simulink model "experiment_toplevel"  (R2016a)
settings: Solver=ode15s  StartTime=0.0  StopTime=20  MaxStep=1e-2  RelTol=1e-4
PreLoadFcn:
  | minitaurParameters
values from neighbouring files (symbols this model uses):
  angular_ctrl_d = 1    [minitaurParameters.m]
  angular_ctrl_i = 1    [minitaurParameters.m]
  angular_ctrl_p = 100    [minitaurParameters.m]
  enc_zero_IA = -1.25*pi    (= -3.92699081699)    [minitaurParameters.m]
  enc_zero_IB = -0.25*pi    (= -0.785398163397)    [minitaurParameters.m]
  enc_zero_IIA = 1.25*pi    (= 3.92699081699)    [minitaurParameters.m]
  enc_zero_IIB = 1.25*pi    (= 3.92699081699)    [minitaurParameters.m]
  enc_zero_IIIA = 0.5*pi    (= 1.57079632679)    [minitaurParameters.m]
  enc_zero_IIIB = 1.5*pi    (= 4.71238898038)    [minitaurParameters.m]
  enc_zero_IVA = -0.25*pi    (= -0.785398163397)    [minitaurParameters.m]
  enc_zero_IVB = 0.5*pi    (= 1.57079632679)    [minitaurParameters.m]
  fore_lag = fore_lag_vals(j)    [experiment1.m]    (also in experiment1_parfor_accelerator.m = 0; minitaurParameters.m = 0.45)
  ground_frame_depth = 0.5    [minitaurParameters.m]
  ground_length = 100    [minitaurParameters.m]
  ground_width = 10    [minitaurParameters.m]
  init_theta_IA = -pi/4    (= -0.785398163397)    [minitaurParameters.m]
  init_theta_IB = pi/4    (= 0.785398163397)    [minitaurParameters.m]
  init_theta_IIA = -pi/4    (= -0.785398163397)    [minitaurParameters.m]
  init_theta_IIB = pi/4    (= 0.785398163397)    [minitaurParameters.m]
  init_theta_IIIA = -pi/4    (= -0.785398163397)    [minitaurParameters.m]
  init_theta_IIIB = pi/4    (= 0.785398163397)    [minitaurParameters.m]
  init_theta_IVA = -pi/4    (= -0.785398163397)    [minitaurParameters.m]
  init_theta_IVB = pi/4    (= 0.785398163397)    [minitaurParameters.m]
  l1 = 100e-3    (= 0.1)    [minitaurParameters.m]
  l2 = 200e-3    (= 0.2)    [minitaurParameters.m]
  leg_joint_radius = 3e-3    (= 0.003)    [minitaurParameters.m]
  lr_sync = 1    [experiment1.m]    (also in experiment1_parfor_accelerator.m; minitaurParameters.m = 0)
  model = 'experiment_toplevel'    [experiment1_parfor_accelerator.m]
  period = period_vals(i)    [experiment1.m]    (also in experiment1_parfor_accelerator.m = 1.5; minitaurParameters.m = 0.33)
  phi_0 = 0.5*asin(l1/l2)    [experiment1.m]    (also in experiment1_parfor_accelerator.m; minitaurParameters.m)
  r_0 = l2    [experiment1.m]    (also in experiment1_parfor_accelerator.m; minitaurParameters.m = 0.2)
  r_x = 0.3*l1    [experiment1.m]    (also in experiment1_parfor_accelerator.m = 0.5*l1; minitaurParameters.m = 0.05)
  r_y = 0.2*l1    [experiment1.m]    (also in experiment1_parfor_accelerator.m = 0.3*l1; minitaurParameters.m = 0.03)
  radial_ctrl_d = 1    [minitaurParameters.m]
  radial_ctrl_i = 1    [minitaurParameters.m]
  radial_ctrl_p = 80    [minitaurParameters.m]
  safety_limit = 10e-3    (= 0.01)    [minitaurParameters.m]
undefined symbols (not defined in the file or in its folder): Axis, Fn, minitaurParams, r_stance, r_swing, stance_frac, X, Y, Z
undefined symbols (not defined in the file): leg_joint_fric_bw, leg_joint_mu_k, leg_joint_mu_s, leg_joint_vel_thresh, motor_kt, motor_kv, motor_r, motor_torque_sat
libraries: sm_lib x453, fl_lib x132, nesl_utility x31, Contact_Forces_Lib x28, simulink x19
(part 1 of 13)
settings Model: TunableVars=fore_lag,lr_sync,period  TunableVarsStorageClass=Auto,Auto,Auto  TunableVarsTypeQualifier=,,  Creator=Alexander  LastModifiedBy=Joe
settings SolverCC: MaxOrder=3  AlgebraicLoopSolver=LineSearch
settings DataIOCC: SaveFormat=StructureWithTime  SaveOutput=off  DSMLogging=off  SaveTime=off  SignalLoggingName=output
settings OptimizationCC: DefaultParameterBehavior=Inlined  InlineInvariantSignals=on  EfficientFloat2IntCast=on  EfficientMapNaN2IntZero=off  AccelVerboseBuild=on
settings DebuggingCC: ReadBeforeWriteMsg=DisableAll  WriteAfterWriteMsg=DisableAll  WriteAfterReadMsg=DisableAll  MultiTaskDSMMsg=none  StrictBusMsg=ErrorOnBusTreatedAsVector
settings HardwareCC: TargetBitPerPointer=64  TargetLongLongMode=on  TargetIntDivRoundTo=Zero  TargetEndianess=LittleEndian  TargetWordSize=64  TargetHWDeviceType=MATLAB Host  ProdEqTarget=off
settings ModelReferenceCC: UpdateModelReferenceTargets=IfOutOfDate  ModelReferenceMinAlgLoopOccurrences=on
settings SFSimCC: SFSimEcho=off  SimBuildMode=sf_nonincremental_build
settings RTWCC: SystemTargetFile=rsim.tlc  TemplateMakefile=rsim_default_tmf  Description=Rapid Simulation Target  Toolchain=MinGW64 v4.x | gmake (64-bit Windows)
settings CodeAppCC: GenerateComments=off  SimulinkBlockComments=off
settings RSimTargetCC: ERTMultiwordTypeDef=System defined  ERTMultiwordLength=256  ConcurrentExecutionCompliant=off  GeneratePreprocessorConditionals=Use local settings  SupportNonFinite=off
settings DiagnosticsConfigSet: SimMechanicsRigidlyBoundBlock=none
settings ExplorerConfigSet: InternalSimMechanicsExplorerSettings="<ExplorerConfiguration><canonicalview>default</canonicalview><AnimationSetting><BasePlaybackSpeed>1.0</BasePlaybackSpeed><PlaybackSpeedFactor>0.015625</PlaybackSpeedFactor></AnimationSetting><TilePanel><TileInfo><Tiles Columns=\"1\" Count=\"1\" Rows=\"1\"><Column Left=\"2\" Weight=\"1\"/><Column Left=\"1404\"/><Row Top=\"2\" Weight=\"1\"/><Row Top=\"894\"/><Tile Height=\"1\" Width=\"1\" X=\"0\" Y=\"0\"/></Tiles></TileInfo><SceneInfo><SceneViewer><BGColor><R>1</R><G>1</G><B>1</B></BGColor><Camera><DoPerspective>off</DoPerspective><Position><X>51.2033483715938971</X><Y>-47.1572080477410083</Y><Z>0.726349227559124011</Z></Position><Center><X>-1.27720243625617513e-06</X><Y>-47.1572080477410083</Y><Z>0.726349227559124011</Z></Center><Up><X>-0</X><Y>0</Y><Z>1</Z></Up><ViewLimDist>1</ViewLimDist><YLim>0.527619672638390491</YLim><XLim>0.832360366914244643</XLim></Camera></SceneViewer></SceneInfo></TilePanel><MechEditorPanel><Cameras><Camera><Id>Camera1</Id><Value><Name>Camera1</Name><NativeCamera><PositionKeyframeSet><Keyframe><Time>+0.0000000000000000e+00</Time><Value><X>+1.6016183665152193e+00</X><Y>-4.6009050514178448e+01</Y><Z>+8.6329844289606328e-01</Z></Value></Keyframe></PositionKeyframeSet><CenterKeyframeSet><Keyframe><Time>+0.0000000000000000e+00</Time><Value><X>+4.1998902890613099e-01</X><Y>-4.6399928223387391e+01</Y><Z>+4.9999520687549426e-01</Z></Value></Keyframe></CenterKeyframeSet><UpVectorKeyframeSet><Keyframe><Time>+0.0000000000000000e+00</Time><Value><X>-2.4497970609361264e-01</X><Y>-1.4974251475434000e-01</Y><Z>+9.5789463036251210e-01</Z></Value></Keyframe></UpVectorKeyframeSet></NativeCamera></Value></Camera></Cameras><GfxPanelCameraMap/></MechEditorPanel></ExplorerConfiguration>"

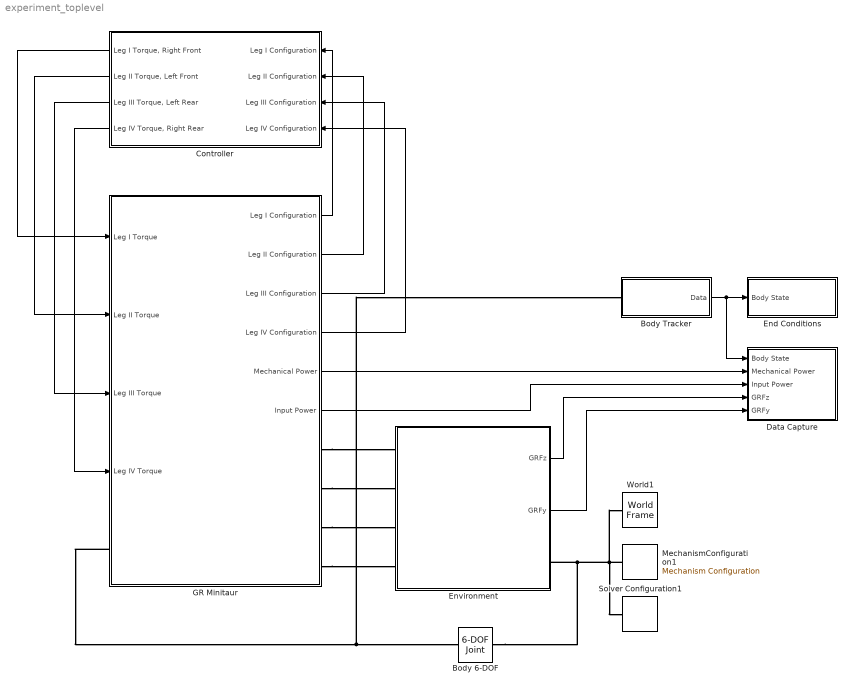
== system experiment_toplevel ==
  Body 6-DOF : sm_lib/Joints/6-DOF Joint  SenseConstraintForce=off  SenseConstraintForceX=off  SenseConstraintForceY=off  SenseConstraintForceZ=off  SenseConstraintTorque=off  SenseConstraintTorqueX=off  SenseConstraintTorqueY=off  SenseConstraintTorqueZ=off  SenseTotalForce=off  SenseTotalForceX=off  SenseTotalForceY=off  SenseTotalForceZ=off  SenseTotalTorque=off  SenseTotalTorqueX=off  SenseTotalTorqueY=off  SenseTotalTorqueZ=off  CompositeWrenchDir=FollowerOnBase  CompositeWrenchFrame=BaseFrame  PxEquilibriumPosition=0  PxEquilibriumPositionUnits=m  PxSpringStiffness=0  PxSpringStiffnessUnits=N/m  PxDampingCoefficient=0  PxDampingCoefficientUnits=N/(m/s)  PxTorqueActuationMode=NoTorque  PxMotionActuationMode=ComputedMotion  PxSensePosition=off  PxSenseVelocity=off  PxSenseAcceleration=off  PxSenseTorqueForce=off  PxPositionTargetSpecify=on  PxPositionTargetPriority=High  PxPositionTargetValue=init_x  PxPositionTargetValueUnits=m  PxVelocityTargetSpecify=off  PxVelocityTargetPriority=High  PxVelocityTargetValue=0  PxVelocityTargetValueUnits=m/s  PyEquilibriumPosition=0  PyEquilibriumPositionUnits=m  PySpringStiffness=0  PySpringStiffnessUnits=N/m  PyDampingCoefficient=0  PyDampingCoefficientUnits=N/(m/s)  PyTorqueActuationMode=NoTorque  PyMotionActuationMode=ComputedMotion  PySensePosition=off  PySenseVelocity=off  PySenseAcceleration=off  PySenseTorqueForce=off  PyPositionTargetSpecify=on  PyPositionTargetPriority=High  PyPositionTargetValue=init_y  PyPositionTargetValueUnits=m  PyVelocityTargetSpecify=off  PyVelocityTargetPriority=High  PyVelocityTargetValue=0  PyVelocityTargetValueUnits=m/s  PzEquilibriumPosition=1  PzEquilibriumPositionUnits=m  PzSpringStiffness=0  PzSpringStiffnessUnits=N/m  PzDampingCoefficient=0  PzDampingCoefficientUnits=N/(m/s)  PzTorqueActuationMode=NoTorque  PzMotionActuationMode=ComputedMotion  PzSensePosition=off  PzSenseVelocity=off  PzSenseAcceleration=off  PzSenseTorqueForce=off  PzPositionTargetSpecify=on  PzPositionTargetPriority=High  PzPositionTargetValue=init_z  PzPositionTargetValueUnits=m  PzVelocityTargetSpecify=off  PzVelocityTargetPriority=High  PzVelocityTargetValue=0  PzVelocityTargetValueUnits=m/s  SphDefPosRotationMethod=None  SphDefPosRotationAngleUnits=deg  SphDefPosRotationStandardAxis=+Z  SphDefPosRotationAngle=0.0  SphDefPosRotationArbitraryAxis=[0 0 1]  SphDefPosFollAlignAxisA=+X  SphDefPosBaseAlignAxisA=+Y  SphDefPosFollAlignAxisB=+Y  SphDefPosBaseAlignAxisB=+Z  SphDefPosRotationSequenceAxes=FollowerAxes  SphDefPosRotationSequence=XYX  SphDefPosRotationSequenceAngles=[0 0 0]  SphDefPosRotationSequenceAnglesUnits=deg  SphDefPosRotationMatrix=[1 0 0; 0 1 0; 0 0 1]  SphEqPosRotationMethod=None  SphEqPosRotationAngleUnits=deg  SphEqPosRotationStandardAxis=+Z  SphEqPosRotationAngle=0.0  SphEqPosRotationArbitraryAxis=[0 0 1]  SphEqPosFollAlignAxisA=+X  SphEqPosBaseAlignAxisA=+Y  SphEqPosFollAlignAxisB=+Y  SphEqPosBaseAlignAxisB=+Z  SphEqPosRotationSequenceAxes=FollowerAxes  SphEqPosRotationSequence=XYX  SphEqPosRotationSequenceAngles=[0 0 0]  SphEqPosRotationSequenceAnglesUnits=deg  SphEqPosRotationMatrix=[1 0 0; 0 1 0; 0 0 1]  SphSpringStiffness=0  SphSpringStiffnessUnits=N*m/deg  SphDampingCoefficient=0  SphDampingCoefficientUnits=N*m/(deg/s)  SphActuateTorqueX=off  SphActuateTorqueY=off  SphActuateTorqueZ=off  SphActuateTorque=off  SphTorqueActuationMode=NoTorque  SphMotionActuationMode=ComputedMotion  SphActuationFrame=BaseFrame  SphSensePosition=off  SphSenseVelocityX=off  SphSenseVelocityY=off  SphSenseVelocityZ=off  SphSenseVelocity=off  SphSenseAccelerationX=off  SphSenseAccelerationY=off  SphSenseAccelerationZ=off  SphSenseAcceleration=off  SphSenseTorqueX=off  SphSenseTorqueY=off  SphSenseTorqueZ=off  SphSenseTorqueForce=off  SphSensingFrame=BaseFrame  SphPositionTargetRotationMethod=RotationSequence  SphPositionTargetRotationAngleUnits=deg  SphPositionTargetRotationStandardAxis=+Z  SphPositionTargetRotationAngle=0.0  SphPositionTargetRotationArbitraryAxis=[0 0 1]  SphPositionTargetFollAlignAxisA=+X  SphPositionTargetBaseAlignAxisA=+Y  SphPositionTargetFollAlignAxisB=+Y  SphPositionTargetBaseAlignAxisB=+Z  SphPositionTargetRotationSequenceAxes=BaseAxes  SphPositionTargetRotationSequence=XZX  SphPositionTargetRotationSequenceAngles=init_rot_xzx  SphPositionTargetRotationSequenceAnglesUnits=deg  SphPositionTargetRotationMatrix=[1 0 0; 0 1 0; 0 0 1]  SphPositionTargetSpecify=on  SphPositionTargetPriority=High  SphVelocityTargetValue=[0 0 0]  SphVelocityTargetValueUnits=deg/s  SphVelocityTargetSpecify=off  SphVelocityTargetPriority=High  SphVelocityTargetInFollowerFrame=on
  Body Tracker : Subsystem
  Controller : Subsystem
  Data Capture : Subsystem
  End Conditions : Subsystem
  Environment : Subsystem
  GR Minitaur : Subsystem
  MechanismConfiguration1 : sm_lib/Utilities/Mechanism Configuration  UniformGravity=Constant  GravityVector="[0  0 -9.81]"  GravityUnits=m/s^2  LinearizationDelta=0.001
  Solver Configuration1 : nesl_utility/Solver Configuration  PhysicalDomain=network_engine_domain  SubClassName=solver  LeftPortType=input  RightPortType=generic  Accelerate=off  Tones=[]  Harmonics=[]  SimulateNoise=off  Profile=off  UseLocalSampling=off  EnableSwitchedLinearOptims=on  FrequencyDomain=off  UseCCode=off  RelTol=0.001  AbsTol=1e-06  MinStep=1e-09  ToWorkspace=off  RevertToSquareIcSolve=off  NumHomotopyIterations=100  PhasorMode=off  PhasorModeNumHarmonics=1  OverrideAbsTol=off  DoDC=off  ResidualTolerance=1e-09  UseLocalSolver=off  LocalSolverChoice=NE_BACKWARD_EULER_ADVANCER  LocalSolverSampleTime=0.001  DoFixedCost=off  MaxNonlinIter=3  MaxModeIter=2  LinearAlgebra=Sparse  DelaysMemoryBudget=1024  AutomaticFiltering=on  FilteringTimeConstant=0.001
  World1 : sm_lib/Frames and Transforms/World Frame
  wires:
  GR Minitaur/1(Leg I Configuration) -> Controller/1(Leg I Configuration)
  GR Minitaur/2(Leg II Configuration) -> Controller/2(Leg II Configuration)
  GR Minitaur/4(Leg IV Configuration) -> Controller/4(Leg IV Configuration)
  Controller/4("Leg IV Torque, Right Rear") -> GR Minitaur/4(Leg IV Torque)
  Controller/3("Leg III Torque, Left Rear") -> GR Minitaur/3(Leg III Torque)
  Controller/2("Leg II Torque, Left Front") -> GR Minitaur/2(Leg II Torque)
  Controller/1("Leg I Torque, Right Front") -> GR Minitaur/1(Leg I Torque)
  Body Tracker/1(Data) -> Data Capture/1(Body State), End Conditions/1(Body State)
  GR Minitaur/5(Mechanical Power) -> Data Capture/2(Mechanical Power)
  GR Minitaur/6(Input Power) -> Data Capture/3(Input Power)
  Environment/1(GRFz) -> Data Capture/4(GRFz)
  Environment/2(GRFy) -> Data Capture/5(GRFy)
  GR Minitaur/3(Leg III Configuration) -> Controller/3(Leg III Configuration)
  connections:
  MechanismConfiguration1/RConn1 -- Solver Configuration1/RConn1 -- Environment/RConn1 -- Body 6-DOF/LConn1 -- World1/RConn1
  GR Minitaur/RConn4 -- Environment/LConn4
  GR Minitaur/RConn3 -- Environment/LConn3
  GR Minitaur/RConn2 -- Environment/LConn2
  GR Minitaur/RConn1 -- Environment/LConn1
  GR Minitaur/LConn1 -- Body Tracker/LConn1 -- Body 6-DOF/RConn1

== system experiment_toplevel/Body Tracker ==
  Mux : Mux  Inputs=6
  PS-Simulink Converter : nesl_utility/PS-Simulink Converter  PhysicalDomain=network_engine_domain  SubClassName=ps_output  LeftPortType=input  RightPortType=output  PseudoPeriodic=off  Frequencies=[]  Unit=m  AffineConversion=off
  PS-Simulink Converter1 : nesl_utility/PS-Simulink Converter  PhysicalDomain=network_engine_domain  SubClassName=ps_output  LeftPortType=input  RightPortType=output  PseudoPeriodic=off  Frequencies=[]  Unit=m  AffineConversion=off
  PS-Simulink Converter2 : nesl_utility/PS-Simulink Converter  PhysicalDomain=network_engine_domain  SubClassName=ps_output  LeftPortType=input  RightPortType=output  PseudoPeriodic=off  Frequencies=[]  Unit=m  AffineConversion=off
  PS-Simulink Converter3 : nesl_utility/PS-Simulink Converter  PhysicalDomain=network_engine_domain  SubClassName=ps_output  LeftPortType=input  RightPortType=output  PseudoPeriodic=off  Frequencies=[]  Unit=m/s  AffineConversion=off
  PS-Simulink Converter4 : nesl_utility/PS-Simulink Converter  PhysicalDomain=network_engine_domain  SubClassName=ps_output  LeftPortType=input  RightPortType=output  PseudoPeriodic=off  Frequencies=[]  Unit=m/s  AffineConversion=off
  PS-Simulink Converter5 : nesl_utility/PS-Simulink Converter  PhysicalDomain=network_engine_domain  SubClassName=ps_output  LeftPortType=input  RightPortType=output  PseudoPeriodic=off  Frequencies=[]  Unit=m/s  AffineConversion=off
  Transform Sensor : sm_lib/Frames and Transforms/Transform Sensor  MeasurementFrame=World  SenseAngle=off  SenseAxis=off  SenseAngle1=off  SenseAngle2=off  SenseAngle3=off  SenseQ=off  SenseR=off  SenseOmegaX=off  SenseOmegaY=off  SenseOmegaZ=off  SenseOmega1=off  SenseOmega2=off  SenseOmega3=off  SenseQDot=off  SenseRDot=off  SenseAlphaX=off  SenseAlphaY=off  SenseAlphaZ=off  SenseAlpha1=off  SenseAlpha2=off  SenseAlpha3=off  SenseQDDot=off  SenseRDDot=off  SenseX=on  SenseY=on  SenseZ=on  SenseRad=off  SenseAzim=off  SenseDist=off  SenseInc=off  SenseXDot=on  SenseYDot=on  SenseZDot=on  SenseRadDot=off  SenseAzimDot=off  SenseDistDot=off  SenseIncDot=off  SenseXDDot=off  SenseYDDot=off  SenseZDDot=off  SenseRadDDot=off  SenseAzimDDot=off  SenseDistDDot=off  SenseIncDDot=off
  World Frame : sm_lib/Frames and Transforms/World Frame
  F : PMIOPort  Port=1  Side=Left
  Data : Outport
  wires:
  PS-Simulink Converter5/1 -> Mux/6
  PS-Simulink Converter4/1 -> Mux/5
  PS-Simulink Converter3/1 -> Mux/4
  PS-Simulink Converter2/1 -> Mux/3
  PS-Simulink Converter1/1 -> Mux/2
  PS-Simulink Converter/1 -> Mux/1
  Mux/1 -> Data/1
  connections:
  PS-Simulink Converter1/LConn1 -- Transform Sensor/RConn3
  PS-Simulink Converter5/LConn1 -- Transform Sensor/RConn7
  PS-Simulink Converter4/LConn1 -- Transform Sensor/RConn6
  F/RConn1 -- Transform Sensor/RConn1
  PS-Simulink Converter/LConn1 -- Transform Sensor/RConn2
  Transform Sensor/LConn1 -- World Frame/RConn1
  PS-Simulink Converter2/LConn1 -- Transform Sensor/RConn4
  PS-Simulink Converter3/LConn1 -- Transform Sensor/RConn5

== system experiment_toplevel/Controller ==
  note: PID trajectory following done in leg workspace (foot position) polar coordinates.
      |
      | PID generates "virtual forces" to be applied at the foot, which are then converted
      | to joint torques using the leg jacobian transpose.
  Leg I Configuration : Inport  PortDimensions=2
  Leg II Configuration : Inport  Port=2  PortDimensions=2
  Leg III Configuration : Inport  Port=3  PortDimensions=2
  Leg IV Configuration : Inport  Port=4  PortDimensions=2
  Subsystem1 : Subsystem
  Subsystem2 : Subsystem
  Subsystem3 : Subsystem
  Subsystem5 : Subsystem
  Trajectory Planner : Subsystem
  "Leg I Torque, Right Front" : Outport
  "Leg II Torque, Left Front" : Outport  Port=2
  "Leg III Torque, Left Rear" : Outport  Port=3
  "Leg IV Torque, Right Rear" : Outport  Port=4
  wires:
  Trajectory Planner/1(Foot I Trajectory [alpha r]) -> Subsystem5/1(Path Trajectory)  "[r_ref theta_ref] m rad"
  Leg I Configuration/1 -> Subsystem5/2(Current leg state)  "[theta_AI theta_BI] Nm"
  Subsystem5/1(Leg Torque) -> "Leg I Torque, Right Front"/1
  Trajectory Planner/2(Foot II Trajectory [alpha r]) -> Subsystem1/1(Path Trajectory)
  Trajectory Planner/3(Foot III Trajectory [alpha r]) -> Subsystem2/1(Path Trajectory)
  Trajectory Planner/4(Foot IV Trajectory [alpha r]) -> Subsystem3/1(Path Trajectory)
  Leg II Configuration/1 -> Subsystem1/2(Current leg state)  "[Tau_IIA Tau_IIB] Nm"
  Leg III Configuration/1 -> Subsystem2/2(Current leg state)  "[Tau_IIIA Tau_IIIB] Nm"
  Leg IV Configuration/1 -> Subsystem3/2(Current leg state)  "[Tau_IVA Tau_IVB] Nm"
  Subsystem1/1(Leg Torque) -> "Leg II Torque, Left Front"/1
  Subsystem2/1(Leg Torque) -> "Leg III Torque, Left Rear"/1
  Subsystem3/1(Leg Torque) -> "Leg IV Torque, Right Rear"/1

== system experiment_toplevel/Data Capture ==
  Body State : Inport
  Mechanical Power : Inport  Port=2
  Input Power : Inport  Port=3
  GRFz : Inport  Port=4
  GRFy : Inport  Port=5
  To Workspace : ToWorkspace  VariableName=P_mech  SaveFormat=Structure With Time  SampleTime=-1
  To Workspace1 : ToWorkspace  VariableName=body_state  SaveFormat=Structure With Time  SampleTime=-1
  To Workspace2 : ToWorkspace  VariableName=P_in  SaveFormat=Structure With Time  SampleTime=-1
  To Workspace3 : ToWorkspace  VariableName=GRF_z  SaveFormat=Structure With Time  SampleTime=-1
  To Workspace4 : ToWorkspace  VariableName=GRF_y  SaveFormat=Structure With Time  SampleTime=-1
  wires:
  Body State/1 -> To Workspace1/1  "body_state"
  Mechanical Power/1 -> To Workspace/1
  Input Power/1 -> To Workspace2/1
  GRFz/1 -> To Workspace3/1  "GRFz"
  GRFy/1 -> To Workspace4/1  "GRFy"

== system experiment_toplevel/End Conditions ==
  Body State : Inport
  Fcn : Fcn  Expr=u(3)<ground_frame_depth
  Fcn1 : Fcn  Expr=u(3)>ground_frame_depth+0.6
  Stop Simulation : Stop
  Stop Simulation1 : Stop
  wires:
  Fcn/1 -> Stop Simulation/1
  Fcn1/1 -> Stop Simulation1/1
  Body State/1 -> Fcn1/1, Fcn/1

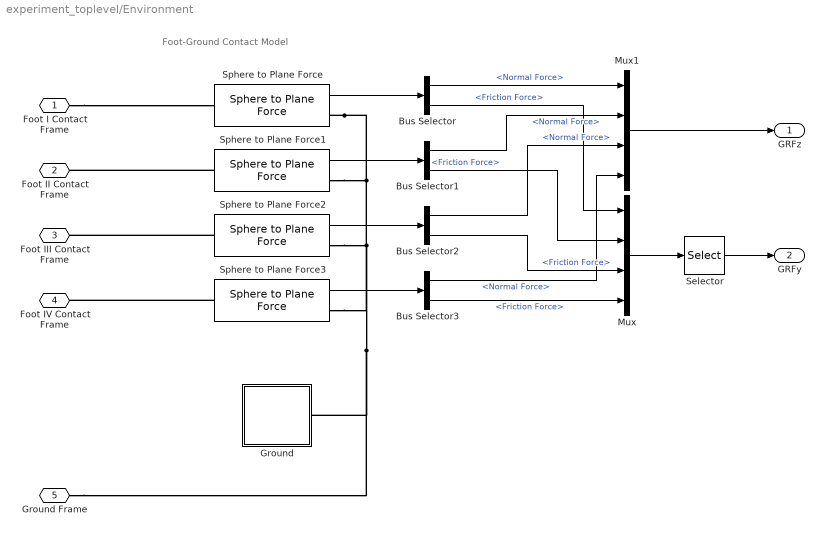
== system experiment_toplevel/Environment ==
  note: Foot-Ground Contact Model
  Bus Selector{,1..3} (4 alike) : BusSelector  OutputSignals=Normal Force,Friction Force
  Ground : Subsystem  mask(Ground (Track) Model){}
      mask help: Models the ground as a rigid body with a given reference frame.
  Mux : Mux
  Mux1 : Mux
  Selector : Selector  IndexMode=Zero-based  InputPortWidth=12  IndexOptions=Index vector (dialog)  Indices=[1:3:11]  OutputSizes=1
  Sphere to Plane Force{,1..3} (4 alike) : Contact_Forces_Lib/3D/Sphere to Plane Force  sphere_rad=foot_contact_radius  plane_lenx=ground_width  plane_leny=ground_length  plane_depth=ground_frame_depth  force_law=Linear  k_contact=foot_contact_stiffness  b_contact=foot_contact_damping  pen_full_damp_F=1e-4  pen_exponent=1  custom_param_1=1  custom_param_2=1  friction_law=Stick-Slip Continuous  mu_kinetic=foot_contact_mu_k  mu_static=foot_contact_mu_s  v_thr=foot_contact_vel_thresh  vis_on=off  vis_opc_en=0  vis_len_plaBz=0.005  vis_clr=[0.9 0.2 0.2]  vis_opc=0.7
  Foot I Contact Frame : PMIOPort  Port=1  Side=Left
  Foot II Contact Frame : PMIOPort  Port=2  Side=Left
  Foot III Contact Frame : PMIOPort  Port=3  Side=Left
  Foot IV Contact Frame : PMIOPort  Port=4  Side=Left
  Ground Frame : PMIOPort  Port=5  Side=Right
  GRFz : Outport
  GRFy : Outport  Port=2
  wires:
  Sphere to Plane Force3/1 -> Bus Selector3/1
  Sphere to Plane Force/1 -> Bus Selector/1
  Sphere to Plane Force1/1 -> Bus Selector1/1
  Sphere to Plane Force2/1 -> Bus Selector2/1
  Bus Selector/1 -> Mux1/1  "<Normal Force>"
  Bus Selector/2 -> Mux/1  "<Friction Force>"
  Bus Selector1/1 -> Mux1/2  "<Normal Force>"
  Bus Selector1/2 -> Mux/2  "<Friction Force>"
  Bus Selector2/1 -> Mux1/3  "<Normal Force>"
  Bus Selector2/2 -> Mux/3  "<Friction Force>"
  Bus Selector3/1 -> Mux1/4  "<Normal Force>"
  Bus Selector3/2 -> Mux/4  "<Friction Force>"
  Mux1/1 -> GRFz/1
  Mux/1 -> Selector/1
  Selector/1 -> GRFy/1
  connections:
  Sphere to Plane Force/RConn1 -- Sphere to Plane Force1/RConn1 -- Sphere to Plane Force2/RConn1 -- Sphere to Plane Force3/RConn1 -- Ground Frame/RConn1 -- Ground/RConn1
  Foot I Contact Frame/RConn1 -- Sphere to Plane Force/LConn1
  Sphere to Plane Force3/LConn1 -- Foot IV Contact Frame/RConn1
  Sphere to Plane Force2/LConn1 -- Foot III Contact Frame/RConn1
  Sphere to Plane Force1/LConn1 -- Foot II Contact Frame/RConn1

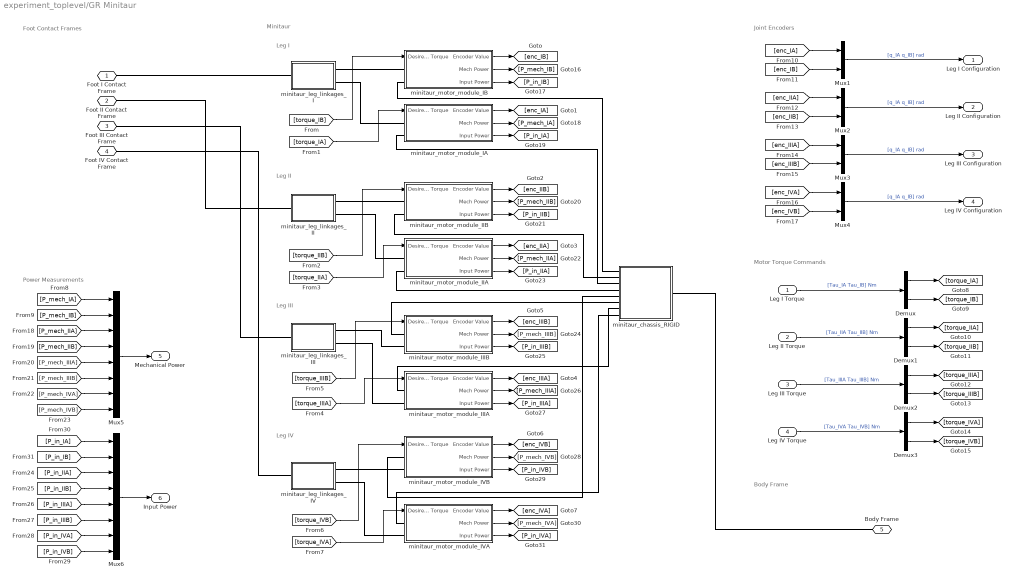
== system experiment_toplevel/GR Minitaur ==
  note: Minitaur
  note: Foot Contact Frames
  note: Joint Encoders
  note: Motor Torque Commands
  note: Body Frame
  note: Power Measurements
  note: Leg I
  note: Leg II
  note: Leg IV
  note: Leg III
  Leg I Torque : Inport
  Leg II Torque : Inport  Port=2
  Leg III Torque : Inport  Port=3
  Leg IV Torque : Inport  Port=4
  Demux{,1..3} (4 alike) : Demux  Outputs=2
  Mux{1..4} (4 alike) : Mux  Inputs=2
  Mux5 : Mux  Inputs=8
  Mux6 : Mux  Inputs=8
  minitaur_chassis_RIGID : Subsystem
  minitaur_leg_linkages_I : Subsystem
  minitaur_leg_linkages_II : Subsystem
  minitaur_leg_linkages_III : Subsystem
  minitaur_leg_linkages_IV : Subsystem
  minitaur_motor_module_IA : Subsystem
  minitaur_motor_module_IB : Subsystem
  minitaur_motor_module_IIA : Subsystem
  minitaur_motor_module_IIB : Subsystem
  minitaur_motor_module_IIIA : Subsystem
  minitaur_motor_module_IIIB : Subsystem
  minitaur_motor_module_IVA : Subsystem
  minitaur_motor_module_IVB : Subsystem
  Foot I Contact Frame : PMIOPort  Port=1  Side=Right
  Foot II Contact Frame : PMIOPort  Port=2  Side=Right
  Foot III Contact Frame : PMIOPort  Port=3  Side=Right
  Foot IV Contact Frame : PMIOPort  Port=4  Side=Right
  Body Frame : PMIOPort  Port=5  Side=Left
  Leg I Configuration : Outport
  Leg II Configuration : Outport  Port=2
  Leg III Configuration : Outport  Port=3
  Leg IV Configuration : Outport  Port=4
  Mechanical Power : Outport  Port=5
  Input Power : Outport  Port=6
  wires:
  Mux1/1 -> Leg I Configuration/1  "[q_IA q_IB] rad"
  Mux2/1 -> Leg II Configuration/1  "[q_IA q_IB] rad"
  Mux3/1 -> Leg III Configuration/1  "[q_IA q_IB] rad"
  Mux4/1 -> Leg IV Configuration/1  "[q_IA q_IB] rad"
  [enc_IB] -> Mux1/2
  [enc_IA] -> Mux1/1
  [enc_IIB] -> Mux2/2
  [enc_IIA] -> Mux2/1
  [enc_IIIB] -> Mux3/2
  [enc_IIIA] -> Mux3/1
  [enc_IVB] -> Mux4/2
  [enc_IVA] -> Mux4/1
  Leg IV Torque/1 -> Demux3/1  "[Tau_IVA Tau_IVB] Nm"
  Leg III Torque/1 -> Demux2/1  "[Tau_IIIA Tau_IIIB] Nm"
  Leg II Torque/1 -> Demux1/1  "[Tau_IIA Tau_IIB] Nm"
  Leg I Torque/1 -> Demux/1  "[Tau_IA Tau_IB] Nm"
  Demux/1 -> [torque_IA]
  Demux/2 -> [torque_IB]
  Demux1/1 -> [torque_IIA]
  Demux1/2 -> [torque_IIB]
  Demux2/1 -> [torque_IIIA]
  Demux2/2 -> [torque_IIIB]
  Demux3/1 -> [torque_IVA]
  Demux3/2 -> [torque_IVB]
  [P_mech_IB] -> Mux5/2
  [P_mech_IA] -> Mux5/1
  [P_mech_IIA] -> Mux5/3
  [P_mech_IIB] -> Mux5/4
  [P_mech_IIIA] -> Mux5/5
  [P_mech_IIIB] -> Mux5/6
  [P_mech_IVA] -> Mux5/7
  [P_mech_IVB] -> Mux5/8
  Mux5/1 -> Mechanical Power/1
  [P_in_IB] -> Mux6/2
  [P_in_IA] -> Mux6/1
  [P_in_IIA] -> Mux6/3
  [P_in_IIB] -> Mux6/4
  [P_in_IIIA] -> Mux6/5
  [P_in_IIIB] -> Mux6/6
  [P_in_IVA] -> Mux6/7
  [P_in_IVB] -> Mux6/8
  Mux6/1 -> Input Power/1
  minitaur_motor_module_IB/1(Encoder Value) -> [enc_IB]
  minitaur_motor_module_IA/1(Encoder Value) -> [enc_IA]
  [torque_IB] -> minitaur_motor_module_IB/1(Desired Torque)
  [torque_IA] -> minitaur_motor_module_IA/1(Desired Torque)
  minitaur_motor_module_IIB/1(Encoder Value) -> [enc_IIB]
  minitaur_motor_module_IIA/1(Encoder Value) -> [enc_IIA]
  [torque_IIB] -> minitaur_motor_module_IIB/1(Desired Torque)
  [torque_IIA] -> minitaur_motor_module_IIA/1(Desired Torque)
  [torque_IIIA] -> minitaur_motor_module_IIIA/1(Desired Torque)
  [torque_IIIB] -> minitaur_motor_module_IIIB/1(Desired Torque)
  minitaur_motor_module_IIIA/1(Encoder Value) -> [enc_IIIA]
  minitaur_motor_module_IIIB/1(Encoder Value) -> [enc_IIIB]
  [torque_IVA] -> minitaur_motor_module_IVA/1(Desired Torque)
  [torque_IVB] -> minitaur_motor_module_IVB/1(Desired Torque)
  minitaur_motor_module_IVB/1(Encoder Value) -> [enc_IVB]
  minitaur_motor_module_IB/3(Input Power) -> [P_in_IB]
  minitaur_motor_module_IB/2(Mech Power) -> [P_mech_IB]
  minitaur_motor_module_IA/2(Mech Power) -> [P_mech_IA]
  minitaur_motor_module_IA/3(Input Power) -> [P_in_IA]
  minitaur_motor_module_IIB/2(Mech Power) -> [P_mech_IIB]
  minitaur_motor_module_IIB/3(Input Power) -> [P_in_IIB]
  minitaur_motor_module_IIA/2(Mech Power) -> [P_mech_IIA]
  minitaur_motor_module_IIA/3(Input Power) -> [P_in_IIA]
  minitaur_motor_module_IIIB/2(Mech Power) -> [P_mech_IIIB]
  minitaur_motor_module_IIIB/3(Input Power) -> [P_in_IIIB]
  minitaur_motor_module_IIIA/2(Mech Power) -> [P_mech_IIIA]
  minitaur_motor_module_IIIA/3(Input Power) -> [P_in_IIIA]
  minitaur_motor_module_IVB/2(Mech Power) -> [P_mech_IVB]
  minitaur_motor_module_IVB/3(Input Power) -> [P_in_IVB]
  minitaur_motor_module_IVA/1(Encoder Value) -> [enc_IVA]
  minitaur_motor_module_IVA/2(Mech Power) -> [P_mech_IVA]
  minitaur_motor_module_IVA/3(Input Power) -> [P_in_IVA]
  connections:
  Foot II Contact Frame/RConn1 -- minitaur_leg_linkages_II/RConn1
  minitaur_leg_linkages_III/RConn1 -- Foot III Contact Frame/RConn1
  minitaur_chassis_RIGID/LConn8 -- minitaur_motor_module_IVA/LConn1
  minitaur_leg_linkages_I/LConn2 -- minitaur_motor_module_IA/LConn1
  minitaur_leg_linkages_I/LConn1 -- minitaur_motor_module_IB/LConn1
  minitaur_leg_linkages_IV/LConn2 -- minitaur_motor_module_IVA/LConn2
  minitaur_leg_linkages_III/LConn1 -- minitaur_motor_module_IIIB/LConn2
  minitaur_chassis_RIGID/LConn6 -- minitaur_motor_module_IIIB/LConn1
  minitaur_leg_linkages_II/LConn2 -- minitaur_motor_module_IIA/LConn1
  minitaur_leg_linkages_II/LConn1 -- minitaur_motor_module_IIB/LConn1
  minitaur_chassis_RIGID/LConn5 -- minitaur_motor_module_IVB/LConn1
  minitaur_chassis_RIGID/LConn4 -- minitaur_motor_module_IIA/LConn2
  minitaur_chassis_RIGID/LConn3 -- minitaur_motor_module_IA/LConn2
  minitaur_chassis_RIGID/LConn7 -- minitaur_motor_module_IIIA/LConn1
  minitaur_chassis_RIGID/LConn2 -- minitaur_motor_module_IIB/LConn2
  minitaur_chassis_RIGID/LConn1 -- minitaur_motor_module_IB/LConn2
  minitaur_leg_linkages_III/LConn2 -- minitaur_motor_module_IIIA/LConn2
  minitaur_leg_linkages_IV/LConn1 -- minitaur_motor_module_IVB/LConn2
  minitaur_chassis_RIGID/RConn1 -- Body Frame/RConn1
  minitaur_leg_linkages_I/RConn1 -- Foot I Contact Frame/RConn1
  minitaur_leg_linkages_IV/RConn1 -- Foot IV Contact Frame/RConn1

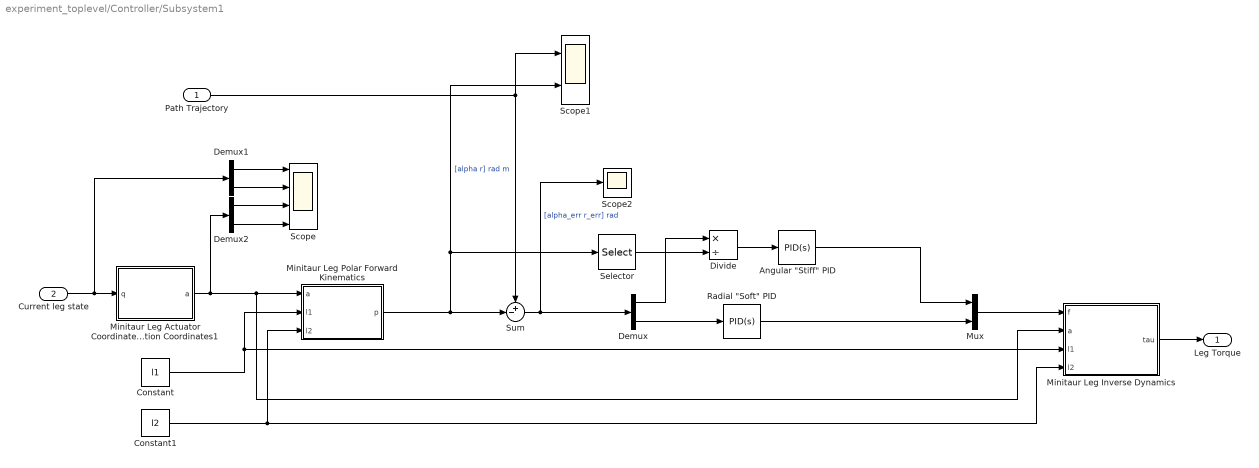
== system experiment_toplevel/Controller/Subsystem1 ==
  Path Trajectory : Inport
  Current leg state : Inport  Port=2
  "Angular \"Stiff\" PID" : simulink/Continuous/PID Controller  Controller=PID  TimeDomain=Continuous-time  SampleTime=-1  IntegratorMethod=Forward Euler  FilterMethod=Forward Euler  Form=Parallel  UseFilter=on  ControllerParametersSource=internal  P=angular_ctrl_p  I=angular_ctrl_i  D=angular_ctrl_d  N=100  InitialConditionSource=internal  InitialConditionForIntegrator=0  InitialConditionForFilter=0  ExternalReset=none  LimitOutput=on  UpperSaturationLimit=inf  LowerSaturationLimit=-inf  LinearizeAsGain=on  AntiWindupMode=clamping  Kb=1  TrackingMode=off  Kt=1  PParamMin=[]  PParamMax=[]  IParamMin=[]  IParamMax=[]  DParamMin=[]  DParamMax=[]  NParamMin=[]  NParamMax=[]  KbParamMin=[]  KbParamMax=[]  KtParamMin=[]  KtParamMax=[]  POutMin=[]  POutMax=[]  IOutMin=[]  IOutMax=[]  DOutMin=[]  DOutMax=[]  NOutMin=[]  NOutMax=[]  KbOutMin=[]  KbOutMax=[]  KtOutMin=[]  KtOutMax=[]  IntegratorOutMin=[]  IntegratorOutMax=[]  FilterOutMin=[]  FilterOutMax=[]  SumOutMin=[]  SumOutMax=[]  SumI1OutMin=[]  SumI1OutMax=[]  SumI2OutMin=[]  SumI2OutMax=[]  SumI3OutMin=[]  SumI3OutMax=[]  SumDOutMin=[]  SumDOutMax=[]  SaturationOutMin=[]  SaturationOutMax=[]  IntegratorContinuousStateAttributes=''  IntegratorStateMustResolveToSignalObject=off  IntegratorRTWStateStorageClass=Auto  FilterContinuousStateAttributes=''  FilterStateMustResolveToSignalObject=off  FilterRTWStateStorageClass=Auto  DifferentiatorICPrevScaledInput=0  DifferentiatorOutMin=[]  DifferentiatorOutMax=[]
  Constant : Constant  Value=l1
  Constant1 : Constant  Value=l2
  Demux : Demux  Outputs=2
  Demux1 : Demux  Outputs=2
  Demux2 : Demux  Outputs=2
  Divide : Product  Inputs=*/
  Minitaur Leg Actuator Coordinates to Configuration Coordinates1 : MATLAB Function  TreatAsAtomicUnit=on
  Minitaur Leg Inverse Dynamics : MATLAB Function  TreatAsAtomicUnit=on
  Minitaur Leg Polar Forward Kinematics : MATLAB Function  TreatAsAtomicUnit=on
  Mux : Mux  Inputs=2
  "Radial \"Soft\" PID" : simulink/Continuous/PID Controller  Controller=PID  TimeDomain=Continuous-time  SampleTime=-1  IntegratorMethod=Forward Euler  FilterMethod=Forward Euler  Form=Parallel  UseFilter=on  ControllerParametersSource=internal  P=radial_ctrl_p  I=radial_ctrl_i  D=radial_ctrl_d  N=100  InitialConditionSource=internal  InitialConditionForIntegrator=0  InitialConditionForFilter=0  ExternalReset=none  LimitOutput=on  UpperSaturationLimit=inf  LowerSaturationLimit=-inf  LinearizeAsGain=on  AntiWindupMode=clamping  Kb=1  TrackingMode=off  Kt=1  PParamMin=[]  PParamMax=[]  IParamMin=[]  IParamMax=[]  DParamMin=[]  DParamMax=[]  NParamMin=[]  NParamMax=[]  KbParamMin=[]  KbParamMax=[]  KtParamMin=[]  KtParamMax=[]  POutMin=[]  POutMax=[]  IOutMin=[]  IOutMax=[]  DOutMin=[]  DOutMax=[]  NOutMin=[]  NOutMax=[]  KbOutMin=[]  KbOutMax=[]  KtOutMin=[]  KtOutMax=[]  IntegratorOutMin=[]  IntegratorOutMax=[]  FilterOutMin=[]  FilterOutMax=[]  SumOutMin=[]  SumOutMax=[]  SumI1OutMin=[]  SumI1OutMax=[]  SumI2OutMin=[]  SumI2OutMax=[]  SumI3OutMin=[]  SumI3OutMax=[]  SumDOutMin=[]  SumDOutMax=[]  SaturationOutMin=[]  SaturationOutMax=[]  IntegratorContinuousStateAttributes=''  IntegratorStateMustResolveToSignalObject=off  IntegratorRTWStateStorageClass=Auto  FilterContinuousStateAttributes=''  FilterStateMustResolveToSignalObject=off  FilterRTWStateStorageClass=Auto  DifferentiatorICPrevScaledInput=0  DifferentiatorOutMin=[]  DifferentiatorOutMax=[]
  Scope : Scope  NumInputPorts=4
  Scope1 : Scope  NumInputPorts=2
  Scope2 : Scope
  Selector : Selector  IndexMode=Zero-based  InputPortWidth=2  IndexOptions=Index vector (dialog)  Indices=[1]  OutputSizes=1
  Sum : Sum  Inputs=+-|
  Leg Torque : Outport
  wires:
  Path Trajectory/1 -> Scope1/1, Sum/1
  Current leg state/1 -> Minitaur Leg Actuator Coordinates to Configuration Coordinates1/1(q), Demux1/1
  Sum/1 -> Demux/1, Scope2/1  "[alpha_err r_err] rad"
  Minitaur Leg Actuator Coordinates to Configuration Coordinates1/1(a) -> Demux2/1, Minitaur Leg Inverse Dynamics/2(a), Minitaur Leg Polar Forward Kinematics/1(a)
  Minitaur Leg Polar Forward Kinematics/1(p) -> Scope1/2, Selector/1, Sum/2  "[alpha r] rad m"
  Demux/2 -> "Radial \"Soft\" PID"/1
  Mux/1 -> Minitaur Leg Inverse Dynamics/1(f)
  Minitaur Leg Inverse Dynamics/1(tau) -> Leg Torque/1
  Constant/1 -> Minitaur Leg Inverse Dynamics/3(l1), Minitaur Leg Polar Forward Kinematics/2(l1)
  Constant1/1 -> Minitaur Leg Inverse Dynamics/4(l2), Minitaur Leg Polar Forward Kinematics/3(l2)
  Demux1/1 -> Scope/1
  Demux1/2 -> Scope/2
  Demux2/1 -> Scope/3
  Demux2/2 -> Scope/4
  Divide/1 -> "Angular \"Stiff\" PID"/1
  Demux/1 -> Divide/1
  Selector/1 -> Divide/2
  "Angular \"Stiff\" PID"/1 -> Mux/1
  "Radial \"Soft\" PID"/1 -> Mux/2

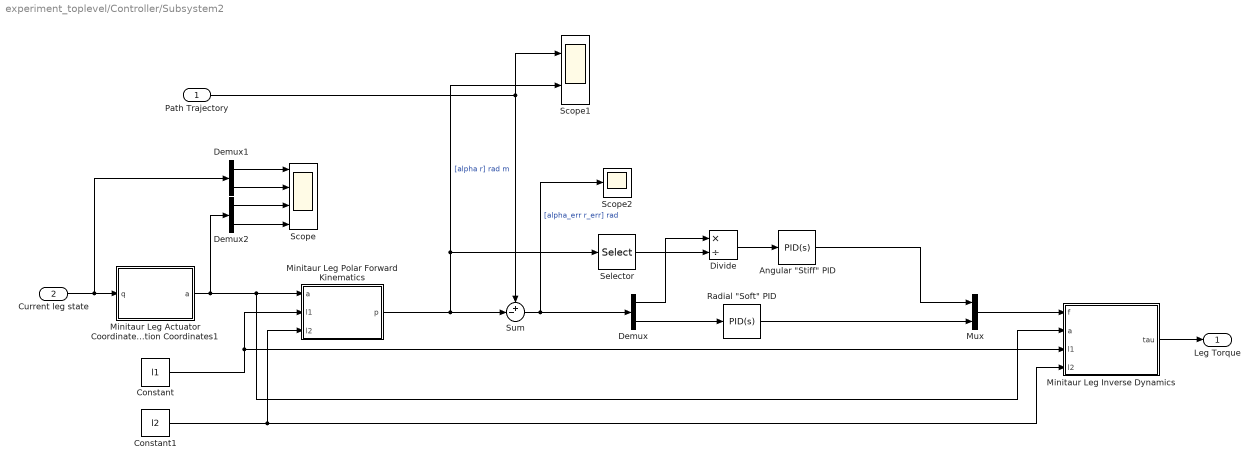
== system experiment_toplevel/Controller/Subsystem2 ==
  Path Trajectory : Inport
  Current leg state : Inport  Port=2
  "Angular \"Stiff\" PID" : simulink/Continuous/PID Controller  Controller=PID  TimeDomain=Continuous-time  SampleTime=-1  IntegratorMethod=Forward Euler  FilterMethod=Forward Euler  Form=Parallel  UseFilter=on  ControllerParametersSource=internal  P=angular_ctrl_p  I=angular_ctrl_i  D=angular_ctrl_d  N=100  InitialConditionSource=internal  InitialConditionForIntegrator=0  InitialConditionForFilter=0  ExternalReset=none  LimitOutput=on  UpperSaturationLimit=inf  LowerSaturationLimit=-inf  LinearizeAsGain=on  AntiWindupMode=clamping  Kb=1  TrackingMode=off  Kt=1  PParamMin=[]  PParamMax=[]  IParamMin=[]  IParamMax=[]  DParamMin=[]  DParamMax=[]  NParamMin=[]  NParamMax=[]  KbParamMin=[]  KbParamMax=[]  KtParamMin=[]  KtParamMax=[]  POutMin=[]  POutMax=[]  IOutMin=[]  IOutMax=[]  DOutMin=[]  DOutMax=[]  NOutMin=[]  NOutMax=[]  KbOutMin=[]  KbOutMax=[]  KtOutMin=[]  KtOutMax=[]  IntegratorOutMin=[]  IntegratorOutMax=[]  FilterOutMin=[]  FilterOutMax=[]  SumOutMin=[]  SumOutMax=[]  SumI1OutMin=[]  SumI1OutMax=[]  SumI2OutMin=[]  SumI2OutMax=[]  SumI3OutMin=[]  SumI3OutMax=[]  SumDOutMin=[]  SumDOutMax=[]  SaturationOutMin=[]  SaturationOutMax=[]  IntegratorContinuousStateAttributes=''  IntegratorStateMustResolveToSignalObject=off  IntegratorRTWStateStorageClass=Auto  FilterContinuousStateAttributes=''  FilterStateMustResolveToSignalObject=off  FilterRTWStateStorageClass=Auto  DifferentiatorICPrevScaledInput=0  DifferentiatorOutMin=[]  DifferentiatorOutMax=[]
  Constant : Constant  Value=l1
  Constant1 : Constant  Value=l2
  Demux : Demux  Outputs=2
  Demux1 : Demux  Outputs=2
  Demux2 : Demux  Outputs=2
  Divide : Product  Inputs=*/
  Minitaur Leg Actuator Coordinates to Configuration Coordinates1 : MATLAB Function  TreatAsAtomicUnit=on
  Minitaur Leg Inverse Dynamics : MATLAB Function  TreatAsAtomicUnit=on
  Minitaur Leg Polar Forward Kinematics : MATLAB Function  TreatAsAtomicUnit=on
  Mux : Mux  Inputs=2
  "Radial \"Soft\" PID" : simulink/Continuous/PID Controller  Controller=PID  TimeDomain=Continuous-time  SampleTime=-1  IntegratorMethod=Forward Euler  FilterMethod=Forward Euler  Form=Parallel  UseFilter=on  ControllerParametersSource=internal  P=radial_ctrl_p  I=radial_ctrl_i  D=radial_ctrl_d  N=100  InitialConditionSource=internal  InitialConditionForIntegrator=0  InitialConditionForFilter=0  ExternalReset=none  LimitOutput=on  UpperSaturationLimit=inf  LowerSaturationLimit=-inf  LinearizeAsGain=on  AntiWindupMode=clamping  Kb=1  TrackingMode=off  Kt=1  PParamMin=[]  PParamMax=[]  IParamMin=[]  IParamMax=[]  DParamMin=[]  DParamMax=[]  NParamMin=[]  NParamMax=[]  KbParamMin=[]  KbParamMax=[]  KtParamMin=[]  KtParamMax=[]  POutMin=[]  POutMax=[]  IOutMin=[]  IOutMax=[]  DOutMin=[]  DOutMax=[]  NOutMin=[]  NOutMax=[]  KbOutMin=[]  KbOutMax=[]  KtOutMin=[]  KtOutMax=[]  IntegratorOutMin=[]  IntegratorOutMax=[]  FilterOutMin=[]  FilterOutMax=[]  SumOutMin=[]  SumOutMax=[]  SumI1OutMin=[]  SumI1OutMax=[]  SumI2OutMin=[]  SumI2OutMax=[]  SumI3OutMin=[]  SumI3OutMax=[]  SumDOutMin=[]  SumDOutMax=[]  SaturationOutMin=[]  SaturationOutMax=[]  IntegratorContinuousStateAttributes=''  IntegratorStateMustResolveToSignalObject=off  IntegratorRTWStateStorageClass=Auto  FilterContinuousStateAttributes=''  FilterStateMustResolveToSignalObject=off  FilterRTWStateStorageClass=Auto  DifferentiatorICPrevScaledInput=0  DifferentiatorOutMin=[]  DifferentiatorOutMax=[]
  Scope : Scope  NumInputPorts=4
  Scope1 : Scope  NumInputPorts=2
  Scope2 : Scope
  Selector : Selector  IndexMode=Zero-based  InputPortWidth=2  IndexOptions=Index vector (dialog)  Indices=[1]  OutputSizes=1
  Sum : Sum  Inputs=+-|
  Leg Torque : Outport
  wires:
  Path Trajectory/1 -> Scope1/1, Sum/1
  Current leg state/1 -> Minitaur Leg Actuator Coordinates to Configuration Coordinates1/1(q), Demux1/1
  Sum/1 -> Demux/1, Scope2/1  "[alpha_err r_err] rad"
  Minitaur Leg Actuator Coordinates to Configuration Coordinates1/1(a) -> Demux2/1, Minitaur Leg Inverse Dynamics/2(a), Minitaur Leg Polar Forward Kinematics/1(a)
  Minitaur Leg Polar Forward Kinematics/1(p) -> Scope1/2, Selector/1, Sum/2  "[alpha r] rad m"
  Demux/2 -> "Radial \"Soft\" PID"/1
  Mux/1 -> Minitaur Leg Inverse Dynamics/1(f)
  Minitaur Leg Inverse Dynamics/1(tau) -> Leg Torque/1
  Constant/1 -> Minitaur Leg Inverse Dynamics/3(l1), Minitaur Leg Polar Forward Kinematics/2(l1)
  Constant1/1 -> Minitaur Leg Inverse Dynamics/4(l2), Minitaur Leg Polar Forward Kinematics/3(l2)
  Demux1/1 -> Scope/1
  Demux1/2 -> Scope/2
  Demux2/1 -> Scope/3
  Demux2/2 -> Scope/4
  Divide/1 -> "Angular \"Stiff\" PID"/1
  Demux/1 -> Divide/1
  Selector/1 -> Divide/2
  "Angular \"Stiff\" PID"/1 -> Mux/1
  "Radial \"Soft\" PID"/1 -> Mux/2

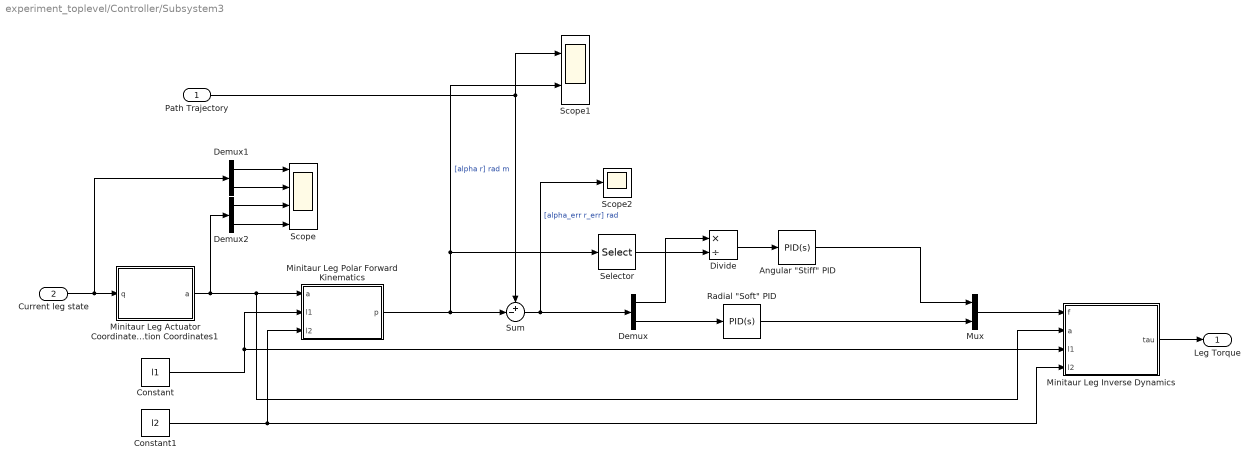
== system experiment_toplevel/Controller/Subsystem3 ==
  Path Trajectory : Inport
  Current leg state : Inport  Port=2
  "Angular \"Stiff\" PID" : simulink/Continuous/PID Controller  Controller=PID  TimeDomain=Continuous-time  SampleTime=-1  IntegratorMethod=Forward Euler  FilterMethod=Forward Euler  Form=Parallel  UseFilter=on  ControllerParametersSource=internal  P=angular_ctrl_p  I=angular_ctrl_i  D=angular_ctrl_d  N=100  InitialConditionSource=internal  InitialConditionForIntegrator=0  InitialConditionForFilter=0  ExternalReset=none  LimitOutput=on  UpperSaturationLimit=inf  LowerSaturationLimit=-inf  LinearizeAsGain=on  AntiWindupMode=clamping  Kb=1  TrackingMode=off  Kt=1  PParamMin=[]  PParamMax=[]  IParamMin=[]  IParamMax=[]  DParamMin=[]  DParamMax=[]  NParamMin=[]  NParamMax=[]  KbParamMin=[]  KbParamMax=[]  KtParamMin=[]  KtParamMax=[]  POutMin=[]  POutMax=[]  IOutMin=[]  IOutMax=[]  DOutMin=[]  DOutMax=[]  NOutMin=[]  NOutMax=[]  KbOutMin=[]  KbOutMax=[]  KtOutMin=[]  KtOutMax=[]  IntegratorOutMin=[]  IntegratorOutMax=[]  FilterOutMin=[]  FilterOutMax=[]  SumOutMin=[]  SumOutMax=[]  SumI1OutMin=[]  SumI1OutMax=[]  SumI2OutMin=[]  SumI2OutMax=[]  SumI3OutMin=[]  SumI3OutMax=[]  SumDOutMin=[]  SumDOutMax=[]  SaturationOutMin=[]  SaturationOutMax=[]  IntegratorContinuousStateAttributes=''  IntegratorStateMustResolveToSignalObject=off  IntegratorRTWStateStorageClass=Auto  FilterContinuousStateAttributes=''  FilterStateMustResolveToSignalObject=off  FilterRTWStateStorageClass=Auto  DifferentiatorICPrevScaledInput=0  DifferentiatorOutMin=[]  DifferentiatorOutMax=[]
  Constant : Constant  Value=l1
  Constant1 : Constant  Value=l2
  Demux : Demux  Outputs=2
  Demux1 : Demux  Outputs=2
  Demux2 : Demux  Outputs=2
  Divide : Product  Inputs=*/
  Minitaur Leg Actuator Coordinates to Configuration Coordinates1 : MATLAB Function  TreatAsAtomicUnit=on
  Minitaur Leg Inverse Dynamics : MATLAB Function  TreatAsAtomicUnit=on
  Minitaur Leg Polar Forward Kinematics : MATLAB Function  TreatAsAtomicUnit=on
  Mux : Mux  Inputs=2
  "Radial \"Soft\" PID" : simulink/Continuous/PID Controller  Controller=PID  TimeDomain=Continuous-time  SampleTime=-1  IntegratorMethod=Forward Euler  FilterMethod=Forward Euler  Form=Parallel  UseFilter=on  ControllerParametersSource=internal  P=radial_ctrl_p  I=radial_ctrl_i  D=radial_ctrl_d  N=100  InitialConditionSource=internal  InitialConditionForIntegrator=0  InitialConditionForFilter=0  ExternalReset=none  LimitOutput=on  UpperSaturationLimit=inf  LowerSaturationLimit=-inf  LinearizeAsGain=on  AntiWindupMode=clamping  Kb=1  TrackingMode=off  Kt=1  PParamMin=[]  PParamMax=[]  IParamMin=[]  IParamMax=[]  DParamMin=[]  DParamMax=[]  NParamMin=[]  NParamMax=[]  KbParamMin=[]  KbParamMax=[]  KtParamMin=[]  KtParamMax=[]  POutMin=[]  POutMax=[]  IOutMin=[]  IOutMax=[]  DOutMin=[]  DOutMax=[]  NOutMin=[]  NOutMax=[]  KbOutMin=[]  KbOutMax=[]  KtOutMin=[]  KtOutMax=[]  IntegratorOutMin=[]  IntegratorOutMax=[]  FilterOutMin=[]  FilterOutMax=[]  SumOutMin=[]  SumOutMax=[]  SumI1OutMin=[]  SumI1OutMax=[]  SumI2OutMin=[]  SumI2OutMax=[]  SumI3OutMin=[]  SumI3OutMax=[]  SumDOutMin=[]  SumDOutMax=[]  SaturationOutMin=[]  SaturationOutMax=[]  IntegratorContinuousStateAttributes=''  IntegratorStateMustResolveToSignalObject=off  IntegratorRTWStateStorageClass=Auto  FilterContinuousStateAttributes=''  FilterStateMustResolveToSignalObject=off  FilterRTWStateStorageClass=Auto  DifferentiatorICPrevScaledInput=0  DifferentiatorOutMin=[]  DifferentiatorOutMax=[]
  Scope : Scope  NumInputPorts=4
  Scope1 : Scope  NumInputPorts=2
  Scope2 : Scope
  Selector : Selector  IndexMode=Zero-based  InputPortWidth=2  IndexOptions=Index vector (dialog)  Indices=[1]  OutputSizes=1
  Sum : Sum  Inputs=+-|
  Leg Torque : Outport
  wires:
  Path Trajectory/1 -> Scope1/1, Sum/1
  Current leg state/1 -> Minitaur Leg Actuator Coordinates to Configuration Coordinates1/1(q), Demux1/1
  Sum/1 -> Demux/1, Scope2/1  "[alpha_err r_err] rad"
  Minitaur Leg Actuator Coordinates to Configuration Coordinates1/1(a) -> Demux2/1, Minitaur Leg Inverse Dynamics/2(a), Minitaur Leg Polar Forward Kinematics/1(a)
  Minitaur Leg Polar Forward Kinematics/1(p) -> Scope1/2, Selector/1, Sum/2  "[alpha r] rad m"
  Demux/2 -> "Radial \"Soft\" PID"/1
  Mux/1 -> Minitaur Leg Inverse Dynamics/1(f)
  Minitaur Leg Inverse Dynamics/1(tau) -> Leg Torque/1
  Constant/1 -> Minitaur Leg Inverse Dynamics/3(l1), Minitaur Leg Polar Forward Kinematics/2(l1)
  Constant1/1 -> Minitaur Leg Inverse Dynamics/4(l2), Minitaur Leg Polar Forward Kinematics/3(l2)
  Demux1/1 -> Scope/1
  Demux1/2 -> Scope/2
  Demux2/1 -> Scope/3
  Demux2/2 -> Scope/4
  Divide/1 -> "Angular \"Stiff\" PID"/1
  Demux/1 -> Divide/1
  Selector/1 -> Divide/2
  "Angular \"Stiff\" PID"/1 -> Mux/1
  "Radial \"Soft\" PID"/1 -> Mux/2

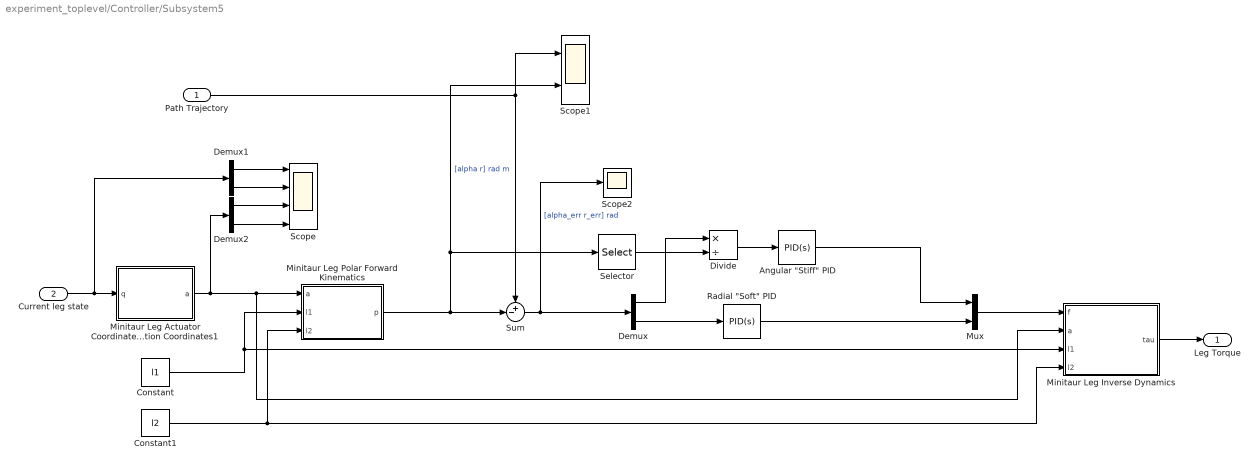
== system experiment_toplevel/Controller/Subsystem5 ==
  Path Trajectory : Inport
  Current leg state : Inport  Port=2
  "Angular \"Stiff\" PID" : simulink/Continuous/PID Controller  Controller=PID  TimeDomain=Continuous-time  SampleTime=-1  IntegratorMethod=Forward Euler  FilterMethod=Forward Euler  Form=Parallel  UseFilter=on  ControllerParametersSource=internal  P=angular_ctrl_p  I=angular_ctrl_i  D=angular_ctrl_d  N=100  InitialConditionSource=internal  InitialConditionForIntegrator=0  InitialConditionForFilter=0  ExternalReset=none  LimitOutput=on  UpperSaturationLimit=inf  LowerSaturationLimit=-inf  LinearizeAsGain=on  AntiWindupMode=clamping  Kb=1  TrackingMode=off  Kt=1  PParamMin=[]  PParamMax=[]  IParamMin=[]  IParamMax=[]  DParamMin=[]  DParamMax=[]  NParamMin=[]  NParamMax=[]  KbParamMin=[]  KbParamMax=[]  KtParamMin=[]  KtParamMax=[]  POutMin=[]  POutMax=[]  IOutMin=[]  IOutMax=[]  DOutMin=[]  DOutMax=[]  NOutMin=[]  NOutMax=[]  KbOutMin=[]  KbOutMax=[]  KtOutMin=[]  KtOutMax=[]  IntegratorOutMin=[]  IntegratorOutMax=[]  FilterOutMin=[]  FilterOutMax=[]  SumOutMin=[]  SumOutMax=[]  SumI1OutMin=[]  SumI1OutMax=[]  SumI2OutMin=[]  SumI2OutMax=[]  SumI3OutMin=[]  SumI3OutMax=[]  SumDOutMin=[]  SumDOutMax=[]  SaturationOutMin=[]  SaturationOutMax=[]  IntegratorContinuousStateAttributes=''  IntegratorStateMustResolveToSignalObject=off  IntegratorRTWStateStorageClass=Auto  FilterContinuousStateAttributes=''  FilterStateMustResolveToSignalObject=off  FilterRTWStateStorageClass=Auto  DifferentiatorICPrevScaledInput=0  DifferentiatorOutMin=[]  DifferentiatorOutMax=[]
  Constant : Constant  Value=l1
  Constant1 : Constant  Value=l2
  Demux : Demux  Outputs=2
  Demux1 : Demux  Outputs=2
  Demux2 : Demux  Outputs=2
  Divide : Product  Inputs=*/
  Minitaur Leg Actuator Coordinates to Configuration Coordinates1 : MATLAB Function  TreatAsAtomicUnit=on
  Minitaur Leg Inverse Dynamics : MATLAB Function  TreatAsAtomicUnit=on
  Minitaur Leg Polar Forward Kinematics : MATLAB Function  TreatAsAtomicUnit=on
  Mux : Mux  Inputs=2
  "Radial \"Soft\" PID" : simulink/Continuous/PID Controller  Controller=PID  TimeDomain=Continuous-time  SampleTime=-1  IntegratorMethod=Forward Euler  FilterMethod=Forward Euler  Form=Parallel  UseFilter=on  ControllerParametersSource=internal  P=radial_ctrl_p  I=radial_ctrl_i  D=radial_ctrl_d  N=100  InitialConditionSource=internal  InitialConditionForIntegrator=0  InitialConditionForFilter=0  ExternalReset=none  LimitOutput=on  UpperSaturationLimit=inf  LowerSaturationLimit=-inf  LinearizeAsGain=on  AntiWindupMode=clamping  Kb=1  TrackingMode=off  Kt=1  PParamMin=[]  PParamMax=[]  IParamMin=[]  IParamMax=[]  DParamMin=[]  DParamMax=[]  NParamMin=[]  NParamMax=[]  KbParamMin=[]  KbParamMax=[]  KtParamMin=[]  KtParamMax=[]  POutMin=[]  POutMax=[]  IOutMin=[]  IOutMax=[]  DOutMin=[]  DOutMax=[]  NOutMin=[]  NOutMax=[]  KbOutMin=[]  KbOutMax=[]  KtOutMin=[]  KtOutMax=[]  IntegratorOutMin=[]  IntegratorOutMax=[]  FilterOutMin=[]  FilterOutMax=[]  SumOutMin=[]  SumOutMax=[]  SumI1OutMin=[]  SumI1OutMax=[]  SumI2OutMin=[]  SumI2OutMax=[]  SumI3OutMin=[]  SumI3OutMax=[]  SumDOutMin=[]  SumDOutMax=[]  SaturationOutMin=[]  SaturationOutMax=[]  IntegratorContinuousStateAttributes=''  IntegratorStateMustResolveToSignalObject=off  IntegratorRTWStateStorageClass=Auto  FilterContinuousStateAttributes=''  FilterStateMustResolveToSignalObject=off  FilterRTWStateStorageClass=Auto  DifferentiatorICPrevScaledInput=0  DifferentiatorOutMin=[]  DifferentiatorOutMax=[]
  Scope : Scope  NumInputPorts=4
  Scope1 : Scope  NumInputPorts=2
  Scope2 : Scope
  Selector : Selector  IndexMode=Zero-based  InputPortWidth=2  IndexOptions=Index vector (dialog)  Indices=[1]  OutputSizes=1
  Sum : Sum  Inputs=+-|
  Leg Torque : Outport
  wires:
  Path Trajectory/1 -> Scope1/1, Sum/1
  Current leg state/1 -> Minitaur Leg Actuator Coordinates to Configuration Coordinates1/1(q), Demux1/1
  Sum/1 -> Demux/1, Scope2/1  "[alpha_err r_err] rad"
  Minitaur Leg Actuator Coordinates to Configuration Coordinates1/1(a) -> Demux2/1, Minitaur Leg Inverse Dynamics/2(a), Minitaur Leg Polar Forward Kinematics/1(a)
  Minitaur Leg Polar Forward Kinematics/1(p) -> Scope1/2, Selector/1, Sum/2  "[alpha r] rad m"
  Demux/2 -> "Radial \"Soft\" PID"/1
  Mux/1 -> Minitaur Leg Inverse Dynamics/1(f)
  Minitaur Leg Inverse Dynamics/1(tau) -> Leg Torque/1
  Constant/1 -> Minitaur Leg Inverse Dynamics/3(l1), Minitaur Leg Polar Forward Kinematics/2(l1)
  Constant1/1 -> Minitaur Leg Inverse Dynamics/4(l2), Minitaur Leg Polar Forward Kinematics/3(l2)
  Demux1/1 -> Scope/1
  Demux1/2 -> Scope/2
  Demux2/1 -> Scope/3
  Demux2/2 -> Scope/4
  Divide/1 -> "Angular \"Stiff\" PID"/1
  Demux/1 -> Divide/1
  Selector/1 -> Divide/2
  "Angular \"Stiff\" PID"/1 -> Mux/1
  "Radial \"Soft\" PID"/1 -> Mux/2
